simulink model "decople2"  (R2020a)
settings: Solver=VariableStepAuto  StartTime=0.0  StopTime=10.0  RelTol=1e-3
values from neighbouring files (symbols this model uses):
  K1 = eval(K)    [decouple2.m]
undefined symbols (not defined in the file or in its folder): A, B, C
settings Model: Creator=wyton  LastModifiedBy=wyton

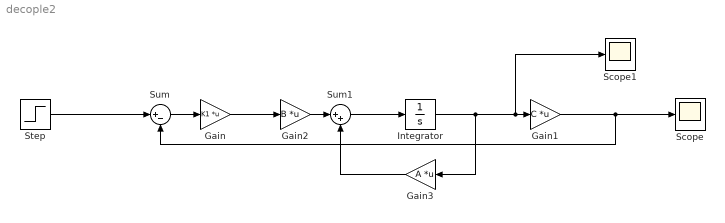
== system decople2 ==
  Gain : Gain  Gain=K1  Multiplication=Matrix(K*u)
  Gain1 : Gain  Gain=C  Multiplication=Matrix(K*u)
  Gain2 : Gain  Gain=B  Multiplication=Matrix(K*u)
  Gain3 : Gain  Gain=A  Multiplication=Matrix(K*u)
  Integrator : Integrator
  Scope : Scope
  Scope1 : Scope
  Step : Step  Before=[0;0]  After=[1;1]  SampleTime=0
  Sum : Sum  Inputs=|+-
  Sum1 : Sum  Inputs=|++
  wires:
  Step/1 -> Sum/1
  Sum/1 -> Gain/1
  Integrator/1 -> Gain3/1, Scope1/1, Gain1/1
  Gain1/1 -> Sum/2, Scope/1
  Sum1/1 -> Integrator/1
  Gain2/1 -> Sum1/1
  Gain3/1 -> Sum1/2
  Gain/1 -> Gain2/1
